simulink model "Five_Truck_Platoon_TS2020"  (Simulink 7.9)
settings: Solver=ode45  StartTime=0.0  StopTime=45  RelTol=1e-3
libraries: Solver_SF x5
settings Model: Creator=elowe  LastModifiedBy=elowe

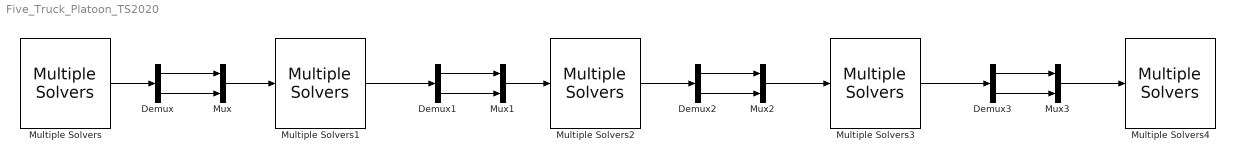
== system Five_Truck_Platoon_TS2020 ==
  Demux{,1..3} (4 alike) : Demux  Outputs=2
  Multiple Solvers : Solver_SF/Multiple Solvers  Priority=1  iVehicle=1  SIMFILE=D:\mech_sim\trunk\Image\TruckSim\Core\TruckSim_Data\Extensions\Simulink\Multi_Vehicle\simfile1.sim  Run_RTs=off  vs_state_ind=Run  StopMode_ind=Vehicle Model  vs_scx=on
  Multiple Solvers1 : Solver_SF/Multiple Solvers  Priority=1  iVehicle=2  SIMFILE=D:\mech_sim\trunk\Image\TruckSim\Core\TruckSim_Data\Extensions\Simulink\Multi_Vehicle\simfile2.sim  Run_RTs=off  vs_state_ind=Run  StopMode_ind=Vehicle Model  vs_scx=on
  Multiple Solvers2 : Solver_SF/Multiple Solvers  Priority=1  iVehicle=3  SIMFILE=D:\mech_sim\trunk\Image\TruckSim\Core\TruckSim_Data\Extensions\Simulink\Multi_Vehicle\simfile3.sim  Run_RTs=off  vs_state_ind=Run  StopMode_ind=Vehicle Model  vs_scx=on
  Multiple Solvers3 : Solver_SF/Multiple Solvers  Priority=1  iVehicle=4  SIMFILE=D:\mech_sim\trunk\Image\TruckSim\Core\TruckSim_Data\Extensions\Simulink\Multi_Vehicle\simfile4.sim  Run_RTs=off  vs_state_ind=Run  StopMode_ind=Vehicle Model  vs_scx=on
  Multiple Solvers4 : Solver_SF/Multiple Solvers  Priority=1  iVehicle=5  SIMFILE=D:\mech_sim\trunk\Image\TruckSim\Core\TruckSim_Data\Extensions\Simulink\Multi_Vehicle\simfile5.sim  Run_RTs=off  vs_state_ind=Run  StopMode_ind=Vehicle Model  vs_scx=on
  Mux{,1..3} (4 alike) : Mux  Inputs=2
  wires:
  Demux/2 -> Mux/2
  Demux/1 -> Mux/1
  Mux/1 -> Multiple Solvers1/1
  Multiple Solvers/1 -> Demux/1
  Demux1/2 -> Mux1/2
  Demux1/1 -> Mux1/1
  Demux2/2 -> Mux2/2
  Demux2/1 -> Mux2/1
  Demux3/2 -> Mux3/2
  Demux3/1 -> Mux3/1
  Multiple Solvers1/1 -> Demux1/1
  Mux1/1 -> Multiple Solvers2/1
  Multiple Solvers2/1 -> Demux2/1
  Mux2/1 -> Multiple Solvers3/1
  Multiple Solvers3/1 -> Demux3/1
  Mux3/1 -> Multiple Solvers4/1
